simulink model "MTQ_Simulation"  (R2024a)
settings: Solver=VariableStepAuto  StartTime=0.0  StopTime=5  RelTol=1e-3
libraries: simulink x1
settings Model: Creator=RAJDEEP PAUL  LastModifiedBy=RAJDEEP PAUL

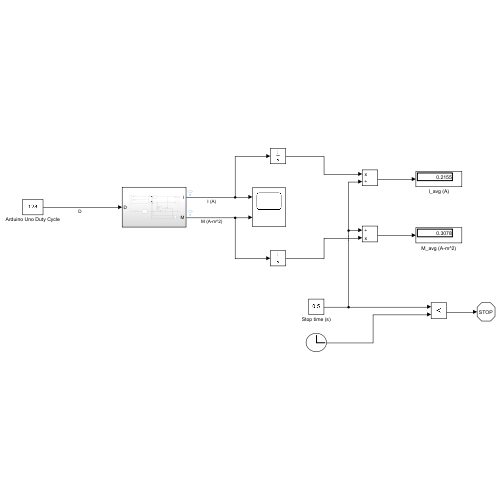
[thumbnail: Simulink's stored preview of the top-level diagram]
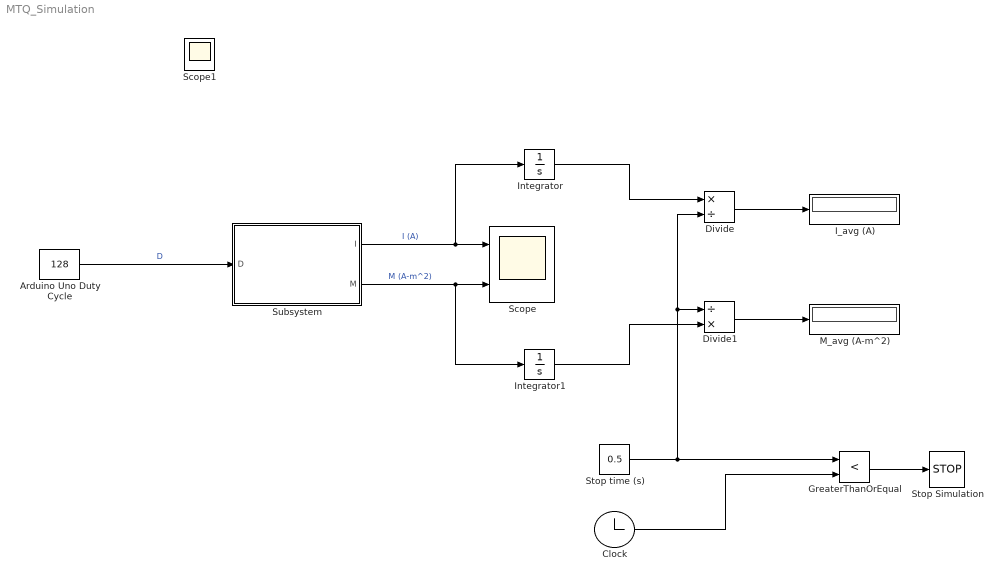
== system MTQ_Simulation ==
  Arduino Uno Duty Cycle : Constant  Value=128
  Clock : Clock
  Divide : Product  Inputs=*/
  Divide1 : Product  Inputs=/*
  GreaterThanOrEqual : RelationalOperator  Operator=<  OutDataTypeStr=boolean  RndMeth=Simplest  InputSameDT=off
  I_avg (A) : Display
  Integrator : Integrator
  Integrator1 : Integrator
  M_avg (A-m^2) : Display
  Scope : Scope  NumInputPorts=2
  Stop Simulation : Stop
  Stop time (s) : Constant  Value=0.5
  Subsystem : Subsystem
  Scope1 : Scope
  wires:
  Integrator/1 -> Divide/1
  Stop time (s)/1 -> Divide/2, Divide1/1, GreaterThanOrEqual/1
  Integrator1/1 -> Divide1/2
  Divide/1 -> I_avg (A)/1
  Divide1/1 -> M_avg (A-m^2)/1
  Clock/1 -> GreaterThanOrEqual/2
  GreaterThanOrEqual/1 -> Stop Simulation/1
  Arduino Uno Duty Cycle/1 -> Subsystem/1(D)  "D"
  Subsystem/1(I) -> Integrator/1, Scope/1  "I (A)"
  Subsystem/2(M) -> Integrator1/1, Scope/2  "M (A-m^2)"

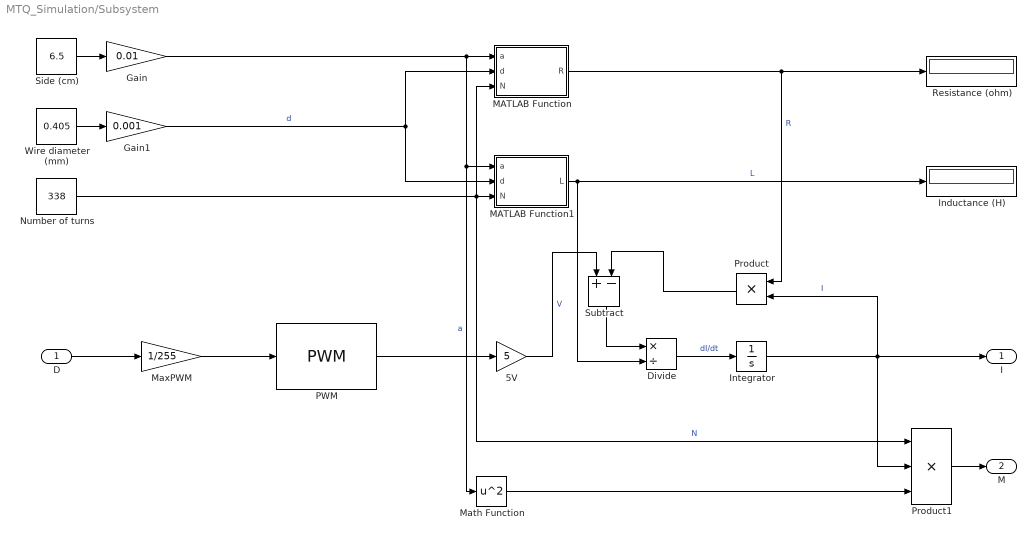
== system MTQ_Simulation/Subsystem ==
  D : Inport
  5V : Gain  Gain=5
  Divide : Product  Inputs=*/
  Gain : Gain  Gain=0.01
  Gain1 : Gain  Gain=0.001
  Inductance (H) : Display
  Integrator : Integrator
  MATLAB Function : MATLAB Function  TreatAsAtomicUnit=on
  MATLAB Function1 : MATLAB Function  TreatAsAtomicUnit=on
  Math Function : Math  Operator=square
  MaxPWM : Gain  Gain=1/255
  Number of turns : Constant  Value=338
  PWM : simulink/Discontinuities/PWM  DisableCoverage=on  Period=1/490  InitialDelay=0  DisallowZeroDutyCycle=off  RunAtFixedTimeIntervals=off  SampleTime=0.1
  Product : Product
  Product1 : Product  Inputs=3
  Resistance (ohm) : Display
  Side (cm) : Constant  Value=6.5
  Subtract : Sum  Inputs=+-
  Wire diameter (mm) : Constant  Value=0.405
  I : Outport
  M : Outport  Port=2
  wires:
  MATLAB Function1/1(L) -> Inductance (H)/1, Divide/2  "L"
  Gain/1 -> MATLAB Function/1(a), MATLAB Function1/1(a), Math Function/1  "a"
  Math Function/1 -> Product1/3
  Product1/1 -> M/1
  Divide/1 -> Integrator/1  "dI/dt"
  Product/1 -> Subtract/2
  MATLAB Function/1(R) -> Resistance (ohm)/1, Product/1  "R"
  Subtract/1 -> Divide/1
  D/1 -> MaxPWM/1
  Number of turns/1 -> Product1/1, MATLAB Function1/3(N), MATLAB Function/3(N)  "N"
  Integrator/1 -> Product1/2, Product/2, I/1  "I"
  5V/1 -> Subtract/1  "V"
  Wire diameter (mm)/1 -> Gain1/1
  MaxPWM/1 -> PWM/1
  PWM/1 -> 5V/1
  Side (cm)/1 -> Gain/1
  Gain1/1 -> MATLAB Function1/2(d), MATLAB Function/2(d)  "d"

== matlab function MTQ_Simulation/Subsystem/MATLAB Function ==
  data: a input; d input; R output; N input
function R = fcn(a, d, N)

l = 4 * a * N;
r = d / 2;
e = 1.7*10^-8;

R = (e * l) / (pi * r^2);

== matlab function MTQ_Simulation/Subsystem/MATLAB Function1 ==
  data: a input; d input; L output; N input
function L = fcn(a, d, N)

r = d / 2;
mu0 = 4 * pi * 10^-7;

L = ((N^2 * 2 * mu0 * a) / pi) * (log(a / r) - 0.774);
